simulink library "myLibrary2019a"  (R2019a)
settings: Solver=VariableStepAuto  StartTime=0.0  StopTime=10.0  RelTol=1e-3
settings Model: Creator=Jesper  LastModifiedBy=Jesper

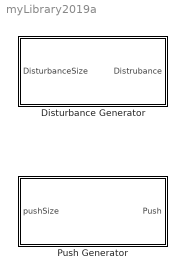
== system myLibrary2019a ==
  Disturbance Generator : Subsystem
  Push Generator : Subsystem  AncestorBlock=myLibrary/Disturbance Generator

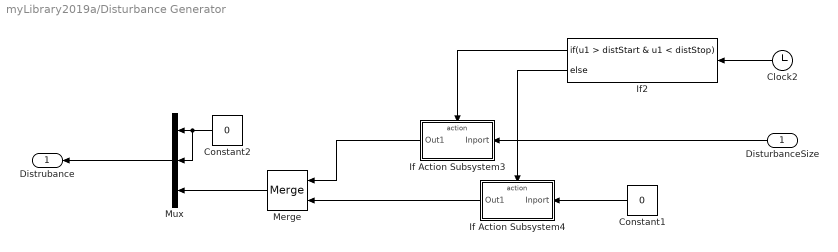
== system myLibrary2019a/Disturbance Generator ==
  DisturbanceSize : Inport
  Clock2 : Clock
  Constant1 : Constant  Value=0
  Constant2 : Constant  Value=0
  If Action Subsystem3 : Subsystem  TreatAsAtomicUnit=on
  If Action Subsystem4 : Subsystem  TreatAsAtomicUnit=on
  If2 : If  IfExpression=u1 > distStart & u1 < distStop
  Merge : Merge
  Mux : Mux  Inputs=3
  Distrubance : Outport
  wires:
  Mux/1 -> Distrubance/1
  If2/2 -> If Action Subsystem4/Action
  Merge/1 -> Mux/3
  If Action Subsystem4/1(Out1) -> Merge/2
  Clock2/1 -> If2/1
  If2/1 -> If Action Subsystem3/Action
  Constant1/1 -> If Action Subsystem4/1(Inport)
  Constant2/1 -> Mux/2, Mux/1
  If Action Subsystem3/1(Out1) -> Merge/1
  DisturbanceSize/1 -> If Action Subsystem3/1(Inport)

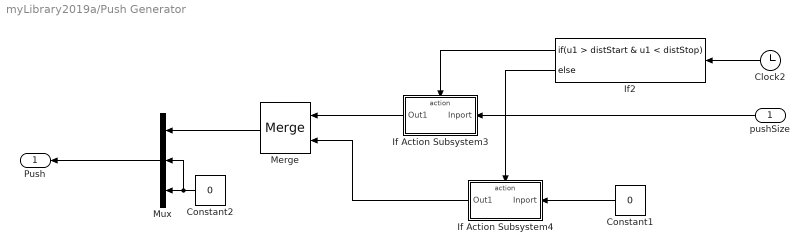
== system myLibrary2019a/Push Generator ==
  pushSize : Inport
  Clock2 : Clock
  Constant1 : Constant  Value=0
  Constant2 : Constant  Value=0
  If Action Subsystem3 : Subsystem  TreatAsAtomicUnit=on
  If Action Subsystem4 : Subsystem  TreatAsAtomicUnit=on
  If2 : If  IfExpression=u1 > distStart & u1 < distStop
  Merge : Merge
  Mux : Mux  Inputs=3
  "Push " : Outport
  wires:
  Mux/1 -> "Push "/1
  If2/2 -> If Action Subsystem4/Action
  If Action Subsystem4/1(Out1) -> Merge/2
  Clock2/1 -> If2/1
  If2/1 -> If Action Subsystem3/Action
  Constant1/1 -> If Action Subsystem4/1(Inport)
  If Action Subsystem3/1(Out1) -> Merge/1
  pushSize/1 -> If Action Subsystem3/1(Inport)
  Constant2/1 -> Mux/2, Mux/3
  Merge/1 -> Mux/1

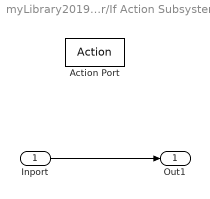
== system myLibrary2019a/Disturbance Generator/If Action Subsystem3 ==
  Inport : Inport
  Action Port : ActionPort
  Out1 : Outport  InitialOutput=0
  wires:
  Inport/1 -> Out1/1

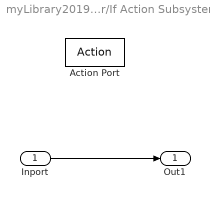
== system myLibrary2019a/Disturbance Generator/If Action Subsystem4 ==
  Inport : Inport
  Action Port : ActionPort
  Out1 : Outport  InitialOutput=0
  wires:
  Inport/1 -> Out1/1

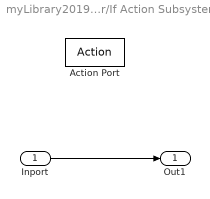
== system myLibrary2019a/Push Generator/If Action Subsystem3 ==
  Inport : Inport
  Action Port : ActionPort
  Out1 : Outport  InitialOutput=0
  wires:
  Inport/1 -> Out1/1

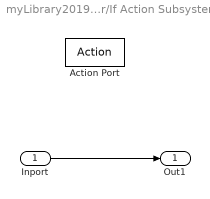
== system myLibrary2019a/Push Generator/If Action Subsystem4 ==
  Inport : Inport
  Action Port : ActionPort
  Out1 : Outport  InitialOutput=0
  wires:
  Inport/1 -> Out1/1
